simulink model "RBDmodel_io"  (R2023a)
settings: Solver=ode15s  StartTime=0.0  StopTime=10  FixedStep=0.0001  RelTol=1e-3  AbsTol=1e-3  EnableMultiTasking=on
model workspace (MAT data in the model file):
  C_Gimbal_FIXED = 0.1
  C_IAP_FIXED = 0.01
  IAP_Pa = 0
  K_Gimbal_FIXED = 0
  K_IAP_FIXED = 0
  Left_EO = 0
  Left_IO = 0
  Left_MF = 0
  Left_RA = 0
  Moment_AR = 0
  Moment_FE = 7.5
  Moment_LB = 0
  Right_EO = 0
  Right_IO = 0
  Right_MF = 0
  Right_RA = 0
  a_FIXED = 1
  b_FIXED = 1
  muscle_color_FIXED = [0 0 1]
  muscle_radius_FIXED = 1
libraries: checkpacklib x3, simulink x1
(part 2 of 2)

== system RBDmodel_io/Model_Outputs/L4-L5 LB readings ==
  L4-L5 LB Simscape Rotation : Inport
  L4-L5 LB Simscape Moment : Inport  Port=2
  L4-L5 LB Moment : Scope
  L4-L5 LB Rotation : Scope
  L4-L5 LB Simscape : Record  FileSettingsInternal="{\"entries\":[{\"content\":{\"excelSettings\":{\"content\":{},\"type\":\"Streamout.ExcelSettings\"}},\"type\":\"Streamout.FileSettingStorage\",\"uuid\":\"9c8fac5d-9f33-464f-a096-b60a5d85e946\"}],\"packageUris\":[\"http://schema.mathworks.com/mf0/streamout_blocks/R2020a\"],\"version\":\"1.0\"}"  Layout=[1 1]  SignalsInternal="{\"entries\":[{\"content\":{\"signals\":[{\"content\":{\"blockPath\":[\"RBDmodel_io/Model_Outputs/L4-L5 LB readings/L4-L5 LB Simscape\"],\"dimensions\":[1],\"domain\":\"RBDmodel_io/Model_Outputs/L4-L5 LB readings/L4-L5 LB Simscape\",\"lineColor\":\"#a2142f\",\"port\":1,\"sid\":[\"\"],\"signalID\":584,\"signalName\":\"L4-L5 LB Simscape Rotation\"},\"type\":\"RecordBlkView.Signal\",\"uuid\":\"747b6cf5-fbd2-464a-8c45-e000cf5d8300\"},{\"content\":{\"blockPath\":[\"RBDmodel_io/Model_Outputs/L4-L5 LB readings/L4-L5 LB Simscape\"],\"dimensions\":[1],\"domain\":\"RBDmodel_io/Model_Outputs/L4-L5 LB readings/L4-L5 LB Simscape\",\"lineColor\":\"#139fff\",\"port\":2,\"sid\":[\"\"],\"signalID\":588,\"signalName\":\"L4-L5 LB Simscape Moment\"},\"type\":\"RecordBlkView.Signal\",\"uuid\":\"a1531055-ee54-45a3-a860-2618397961a4\"}]},\"type\":\"RecordBlkView.InputSignals\",\"uuid\":\"e3305804-3762-4a25-9e33-32075b1a32bf\"}],\"packageUris\":[\"http://schema.mathworks.com/mf0/streamout_blocks/R2020a\"],\"version\":\"1.0\"}"  VisualizationBindings="{\"xyplotplugin\":{\"info\":[{\"series\":[],\"subplotID\":1}]}}"  CompatibilityTag=XY
  wires:
  L4-L5 LB Simscape Moment/1 -> L4-L5 LB Simscape/2, L4-L5 LB Moment/1
  L4-L5 LB Simscape Rotation/1 -> L4-L5 LB Simscape/1, L4-L5 LB Rotation/1

== system RBDmodel_io/Model_Outputs/L5-S1 AR readings ==
  L5-S1 AR Simscape Rotation : Inport
  L5-S1 AR Simscape Moment : Inport  Port=2
  L5-S1 AR Moment : Scope
  L5-S1 AR Rotation : Scope
  L5-S1 AR Simscape : Record  FileSettingsInternal="{\"entries\":[{\"content\":{\"excelSettings\":{\"content\":{},\"type\":\"Streamout.ExcelSettings\"}},\"type\":\"Streamout.FileSettingStorage\",\"uuid\":\"629b0c74-dae5-4a53-9ac1-6e0aa878d695\"}],\"packageUris\":[\"http://schema.mathworks.com/mf0/streamout_blocks/R2020a\"],\"version\":\"1.0\"}"  Layout=[1 1]  SignalsInternal="{\"entries\":[{\"content\":{\"signals\":[{\"content\":{\"blockPath\":[\"RBDmodel_io/Model_Outputs/L5-S1 AR readings/L5-S1 AR Simscape\"],\"dimensions\":[1],\"domain\":\"RBDmodel_io/Model_Outputs/L5-S1 AR readings/L5-S1 AR Simscape\",\"lineColor\":\"#edb120\",\"port\":1,\"sid\":[\"\"],\"signalID\":624,\"signalName\":\"L5-S1 AR Simscape Rotation\"},\"type\":\"RecordBlkView.Signal\",\"uuid\":\"c29fc12f-cf20-4e01-bf70-ce8460c0b9ce\"},{\"content\":{\"blockPath\":[\"RBDmodel_io/Model_Outputs/L5-S1 AR readings/L5-S1 AR Simscape\"],\"dimensions\":[1],\"domain\":\"RBDmodel_io/Model_Outputs/L5-S1 AR readings/L5-S1 AR Simscape\",\"lineColor\":\"#7e2f8e\",\"port\":2,\"sid\":[\"\"],\"signalID\":628,\"signalName\":\"L5-S1 AR Simscape Moment\"},\"type\":\"RecordBlkView.Signal\",\"uuid\":\"057c8e3e-dfb0-4dda-9953-3f9dfca4dbea\"}]},\"type\":\"RecordBlkView.InputSignals\",\"uuid\":\"a138d924-95b2-44e4-ae18-4626f9f3a9e0\"}],\"packageUris\":[\"http://schema.mathworks.com/mf0/streamout_blocks/R2020a\"],\"version\":\"1.0\"}"  VisualizationBindings="{\"xyplotplugin\":{\"info\":[{\"series\":[],\"subplotID\":1}]}}"  CompatibilityTag=XY
  wires:
  L5-S1 AR Simscape Rotation/1 -> L5-S1 AR Simscape/1, L5-S1 AR Rotation/1
  L5-S1 AR Simscape Moment/1 -> L5-S1 AR Simscape/2, L5-S1 AR Moment/1

== system RBDmodel_io/Model_Outputs/L5-S1 FE readings ==
  L5-S1 FE Simscape Rotation : Inport
  L5-S1 FE Simscape Moment : Inport  Port=2
  L5-S1 FE M-R : Record  FileSettingsInternal="{\"entries\":[{\"content\":{\"excelSettings\":{\"content\":{},\"type\":\"Streamout.ExcelSettings\"}},\"type\":\"Streamout.FileSettingStorage\",\"uuid\":\"bdfbc93e-6c60-4ded-934a-2b1317595bda\"}],\"packageUris\":[\"http://schema.mathworks.com/mf0/streamout_blocks/R2020a\"],\"version\":\"1.0\"}"  Layout=[1 1]  SignalsInternal="{\"entries\":[{\"content\":{\"signals\":[{\"content\":{\"blockPath\":[\"RBDmodel_io/Model_Outputs/L5-S1 FE readings/L5-S1 FE M-R\"],\"dimensions\":[1],\"domain\":\"RBDmodel_io/Model_Outputs/L5-S1 FE readings/L5-S1 FE M-R\",\"lineColor\":\"#fe330a\",\"port\":1,\"sid\":[\"\"],\"signalID\":496,\"signalName\":\"L5-S1 FE Simscape Rotation\"},\"type\":\"RecordBlkView.Signal\",\"uuid\":\"3c699a6b-89fc-4402-ae94-5eb35b4fe517\"},{\"content\":{\"blockPath\":[\"RBDmodel_io/Model_Outputs/L5-S1 FE readings/L5-S1 FE M-R\"],\"dimensions\":[1],\"domain\":\"RBDmodel_io/Model_Outputs/L5-S1 FE readings/L5-S1 FE M-R\",\"lineColor\":\"#22b573\",\"port\":2,\"sid\":[\"\"],\"signalID\":500,\"signalName\":\"L5-S1 FE Simscape Moment\"},\"type\":\"RecordBlkView.Signal\",\"uuid\":\"23d2bb5f-1ab1-4bbf-8452-a04058fad9a6\"}]},\"type\":\"RecordBlkView.InputSignals\",\"uuid\":\"3996b656-5dfa-4715-b5e6-396fbade42dc\"}],\"packageUris\":[\"http://schema.mathworks.com/mf0/streamout_blocks/R2020a\"],\"version\":\"1.0\"}"  VisualizationBindings="{\"xyplotplugin\":{\"info\":[{\"series\":[],\"subplotID\":1}]}}"  CompatibilityTag=XY
  L5-S1 FE Moment : Scope
  L5-S1 FE Rot : Scope
  wires:
  L5-S1 FE Simscape Rotation/1 -> L5-S1 FE M-R/1, L5-S1 FE Rot/1
  L5-S1 FE Simscape Moment/1 -> L5-S1 FE M-R/2, L5-S1 FE Moment/1

== system RBDmodel_io/Model_Outputs/L5-S1 LB readings ==
  L5-S1 LB Simscape Rotation : Inport
  L5-S1 LB Simscape Moment : Inport  Port=2
  L5-S1 LB Moment : Scope
  L5-S1 LB Rotation : Scope
  L5-S1 LB Simscape : Record  FileSettingsInternal="{\"entries\":[{\"content\":{\"excelSettings\":{\"content\":{},\"type\":\"Streamout.ExcelSettings\"}},\"type\":\"Streamout.FileSettingStorage\",\"uuid\":\"88792920-b754-4645-a1ab-98fa44608aca\"}],\"packageUris\":[\"http://schema.mathworks.com/mf0/streamout_blocks/R2020a\"],\"version\":\"1.0\"}"  Layout=[1 1]  SignalsInternal="{\"entries\":[{\"content\":{\"signals\":[{\"content\":{\"blockPath\":[\"RBDmodel_io/Model_Outputs/L5-S1 LB readings/L5-S1 LB Simscape\"],\"dimensions\":[1],\"domain\":\"RBDmodel_io/Model_Outputs/L5-S1 LB readings/L5-S1 LB Simscape\",\"lineColor\":\"#77ac30\",\"port\":1,\"sid\":[\"\"],\"signalID\":576,\"signalName\":\"L5-S1 LB Simscape Rotation\"},\"type\":\"RecordBlkView.Signal\",\"uuid\":\"3932d6d2-4dfe-4f54-a827-0093070966a5\"},{\"content\":{\"blockPath\":[\"RBDmodel_io/Model_Outputs/L5-S1 LB readings/L5-S1 LB Simscape\"],\"dimensions\":[1],\"domain\":\"RBDmodel_io/Model_Outputs/L5-S1 LB readings/L5-S1 LB Simscape\",\"lineColor\":\"#4dbeee\",\"port\":2,\"sid\":[\"\"],\"signalID\":580,\"signalName\":\"L5-S1 LB Simscape Moment\"},\"type\":\"RecordBlkView.Signal\",\"uuid\":\"ed273294-4978-4b07-8170-6408fa638fbc\"}]},\"type\":\"RecordBlkView.InputSignals\",\"uuid\":\"32523f99-eedc-46a9-919e-4b9ad9d14562\"}],\"packageUris\":[\"http://schema.mathworks.com/mf0/streamout_blocks/R2020a\"],\"version\":\"1.0\"}"  VisualizationBindings="{\"xyplotplugin\":{\"info\":[{\"series\":[],\"subplotID\":1}]}}"  CompatibilityTag=XY
  wires:
  L5-S1 LB Simscape Moment/1 -> L5-S1 LB Simscape/2, L5-S1 LB Moment/1
  L5-S1 LB Simscape Rotation/1 -> L5-S1 LB Simscape/1, L5-S1 LB Rotation/1

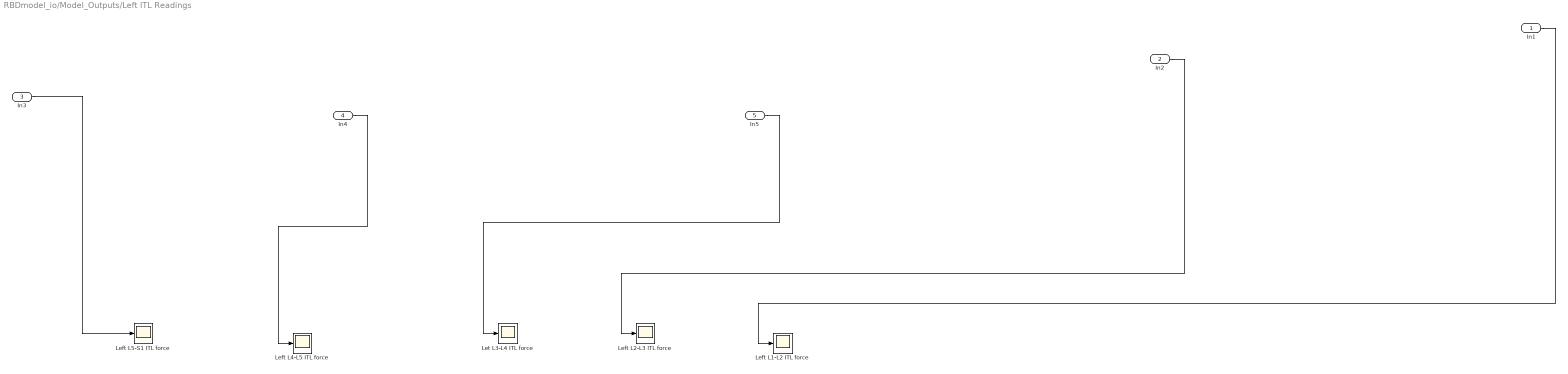
== system RBDmodel_io/Model_Outputs/Left ITL Readings ==
  In1 : Inport
  In2 : Inport  Port=2
  In3 : Inport  Port=3
  In4 : Inport  Port=4
  In5 : Inport  Port=5
  Left L1-L2 ITL force : Scope
  Left L2-L3 ITL force : Scope
  Left L4-L5 ITL force : Scope
  Left L5-S1 ITL force : Scope
  Let L3-L4 ITL force : Scope
  wires:
  In4/1 -> Left L4-L5 ITL force/1
  In1/1 -> Left L1-L2 ITL force/1
  In5/1 -> Let L3-L4 ITL force/1
  In3/1 -> Left L5-S1 ITL force/1
  In2/1 -> Left L2-L3 ITL force/1

== system RBDmodel_io/Model_Outputs/Plumbline readings ==
  x : Inport
  y : Inport  Port=2
  z : Inport  Port=3
  Check X Bounds : checkpacklib/Check Custom Bounds  InstantiateOnLoad=on  enabled=off  stopWhenAssertionFail=off  export=off  ViewDlgPos=[983.4 172.2 510.4 379.2]  OpenViewOnLoad=off  LaunchViewOnOpen=off  TimeUnits=seconds  EnableUpperBound=on  UpperBoundTimes=[0 3]  UpperBoundAmplitudes=[2 2];  EnableLowerBound=on  LowerBoundTimes=[0 3]  LowerBoundAmplitudes=[-2 -2]
      settings: LibrarySourceBlock=sdolib/Signal Constraints/Check Custom Bounds
  Check Y Bounds : checkpacklib/Check Custom Bounds  InstantiateOnLoad=on  enabled=off  stopWhenAssertionFail=off  export=off  ViewDlgPos=[509 222 510 390]  OpenViewOnLoad=off  LaunchViewOnOpen=off  TimeUnits=seconds  EnableUpperBound=on  UpperBoundTimes=[0 3]  UpperBoundAmplitudes=[2 2];  EnableLowerBound=on  LowerBoundTimes=[0 3]  LowerBoundAmplitudes=[-2 -2]
      settings: LibrarySourceBlock=sdolib/Signal Constraints/Check Custom Bounds
  Plumbline X distance (cm) : Display
  Plumbline Y distance (cm) : Display
  Plumbline Z distance (cm) : Display
  T1 plumbline coordinates : Scope  NumInputPorts=3
  wires:
  x/1 -> Plumbline X distance (cm)/1, Check X Bounds/1, T1 plumbline coordinates/1
  z/1 -> Plumbline Z distance (cm)/1, T1 plumbline coordinates/3
  y/1 -> Plumbline Y distance (cm)/1, Check Y Bounds/1, T1 plumbline coordinates/2

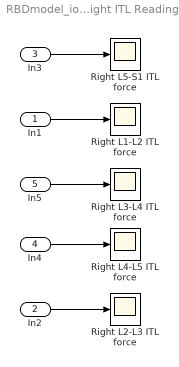
== system RBDmodel_io/Model_Outputs/Right ITL Readings ==
  In1 : Inport
  In2 : Inport  Port=2
  In3 : Inport  Port=3
  In4 : Inport  Port=4
  In5 : Inport  Port=5
  Right L1-L2 ITL force : Scope
  Right L2-L3 ITL force : Scope
  Right L3-L4 ITL force : Scope
  Right L4-L5 ITL force : Scope
  Right L5-S1 ITL force : Scope
  wires:
  In5/1 -> Right L3-L4 ITL force/1
  In1/1 -> Right L1-L2 ITL force/1
  In3/1 -> Right L5-S1 ITL force/1
  In2/1 -> Right L2-L3 ITL force/1
  In4/1 -> Right L4-L5 ITL force/1

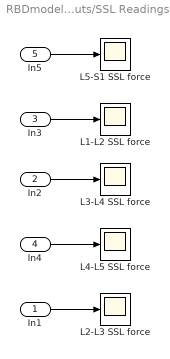
== system RBDmodel_io/Model_Outputs/SSL Readings ==
  In1 : Inport
  In2 : Inport  Port=2
  In3 : Inport  Port=3
  In4 : Inport  Port=4
  In5 : Inport  Port=5
  L1-L2 SSL force : Scope
  L2-L3 SSL force : Scope
  L3-L4 SSL force : Scope
  L4-L5 SSL force : Scope
  L5-S1 SSL force : Scope
  wires:
  In5/1 -> L5-S1 SSL force/1
  In3/1 -> L1-L2 SSL force/1
  In1/1 -> L2-L3 SSL force/1
  In2/1 -> L3-L4 SSL force/1
  In4/1 -> L4-L5 SSL force/1

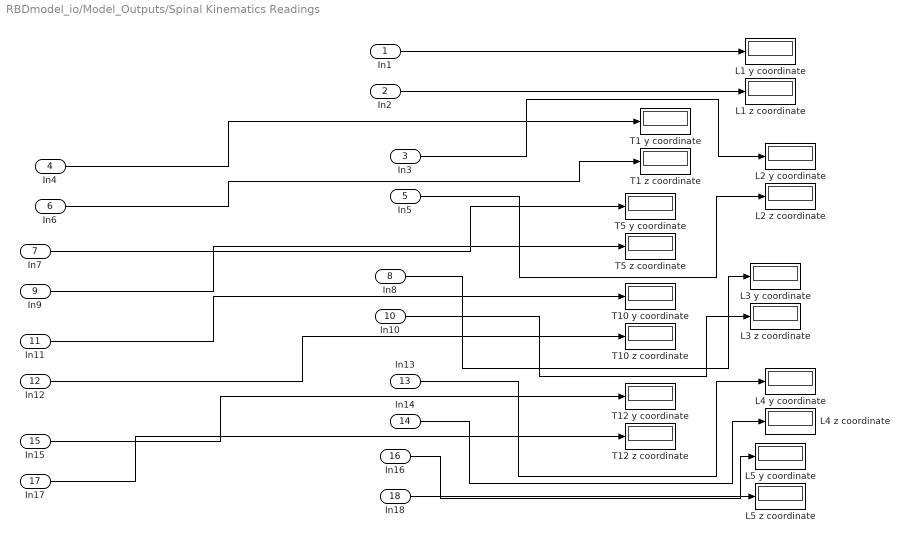
== system RBDmodel_io/Model_Outputs/Spinal Kinematics Readings ==
  In1 : Inport
  In2 : Inport  Port=2
  In3 : Inport  Port=3
  In4 : Inport  Port=4
  In5 : Inport  Port=5
  In6 : Inport  Port=6
  In7 : Inport  Port=7
  In8 : Inport  Port=8
  In9 : Inport  Port=9
  In10 : Inport  Port=10
  In11 : Inport  Port=11
  In12 : Inport  Port=12
  In13 : Inport  Port=13
  In14 : Inport  Port=14
  In15 : Inport  Port=15
  In16 : Inport  Port=16
  In17 : Inport  Port=17
  In18 : Inport  Port=18
  L1 y coordinate : Display
  L1 z coordinate : Display
  L2 y coordinate : Display
  L2 z coordinate : Display
  L3 y coordinate : Display
  L3 z coordinate : Display
  L4 y coordinate : Display
  L4 z coordinate : Display
  L5 y coordinate : Display
  L5 z coordinate : Display
  T1 y coordinate : Display
  T1 z coordinate : Display
  T10 y coordinate : Display
  T10 z coordinate : Display
  T12 y coordinate : Display
  T12 z coordinate : Display
  T5 y coordinate : Display
  T5 z coordinate : Display
  wires:
  In2/1 -> L1 z coordinate/1
  In7/1 -> T5 y coordinate/1
  In13/1 -> L4 y coordinate/1
  In10/1 -> L3 z coordinate/1
  In18/1 -> L5 z coordinate/1
  In6/1 -> T1 z coordinate/1
  In3/1 -> L2 y coordinate/1
  In11/1 -> T10 y coordinate/1
  In9/1 -> T5 z coordinate/1
  In1/1 -> L1 y coordinate/1
  In5/1 -> L2 z coordinate/1
  In14/1 -> L4 z coordinate/1
  In15/1 -> T12 y coordinate/1
  In4/1 -> T1 y coordinate/1
  In12/1 -> T10 z coordinate/1
  In8/1 -> L3 y coordinate/1
  In17/1 -> T12 z coordinate/1
  In16/1 -> L5 y coordinate/1

== matlab function RBDmodel_io/Model_Inputs/Muscle force inputs/Sum of Square of Forces ==
  data: F1 input; SumofSquareofForces output; F2 input; F3 input; F4 input; F5 input; F6 input; F7 input; F8 input; IAP input
function SumofSquareofForces = fcn(F1,F2,F3,F4,F5,F6,F7,F8,IAP)

SumofSquareofForces = F1^2 + F2^2 + F3^2 + F4^2 + F5^2 + F6^2 +F7^2 + F8^2 + IAP^2;
